simulink model "sync_mach_disc_sim"  (R2017a)
settings: Solver=FixedStepAuto  StartTime=0.0  StopTime=10.0  FixedStep=1e-5  RelTol=1e-3
values from neighbouring files (symbols this model uses):
  L_1 = inv(L)    [smparamlib.m]
  Ra = .018    (= 0.018)    [smparamlib.m]
  Rf = 0.001    [smparamlib.m]
  Rkd = 0.02    [smparamlib.m]
  Rkq = 0.04    [smparamlib.m]
  wo = 2*pi*freq0    (= 376.991118431)    [smparamlib.m]
undefined symbols (not defined in the file or in its folder): DiscIntNeverNeededParam
settings Model: Creator=krovchen  LastModifiedBy=krovchen
settings OptimizationCC: DefaultParameterBehavior=Inlined  UseDivisionForNetSlopeComputation=on  UseFloatMulNetSlope=on  InlineInvariantSignals=on  PassReuseOutputArgsAs=Individual arguments  ZeroExternalMemoryAtStartup=off  ZeroInternalMemoryAtStartup=off  NoFixptDivByZeroProtection=on  EfficientFloat2IntCast=on
settings DebuggingCC: ParameterTunabilityLossMsg=error
settings SFSimCC: MATLABDynamicMemAlloc=off
settings RTWCC: SystemTargetFile=ert.tlc  GenCodeOnly=on  GenerateMakefile=off  PackageGeneratedCodeAndArtifacts=on  PackageName=v1_model_export  TemplateMakefile=RTW.MSVCBuild  Description=Create Visual C/C++ Solution File for Embedded Coder  GenerateReport=on  IncludeHyperlinkInReport=on  LaunchReport=on  TargetLang=C++  GenerateTraceInfo=on  GenerateTraceReport=on  GenerateTraceReportSl=on  GenerateTraceReportSf=on  GenerateTraceReportEml=on
settings CodeAppCC: ForceParamTrailComments=on  IgnoreCustomStorageClasses=off  OperatorAnnotations=on  SimulinkDataObjDesc=on  SFDataObjDesc=on  MATLABFcnDesc=on  CustomSymbolStrGlobalVar=rt$N$M  CustomSymbolStrType=$N$M  CustomSymbolStrFcn=$N$M$F  CustomSymbolStrMacro=$N$M  InsertBlockDesc=on  MATLABSourceComments=on
settings ERTTargetCC: TargetLangStandard=C++03 (ISO)  GenerateSampleERTMain=on  MultiInstanceERTCode=on  CodeInterfacePackaging=C++ class  SupportContinuousTime=on  InlinedParameterPlacement=NonHierarchical  RootIOFormat=Structure reference  ERTCustomFileTemplate=example_file_process.tlc

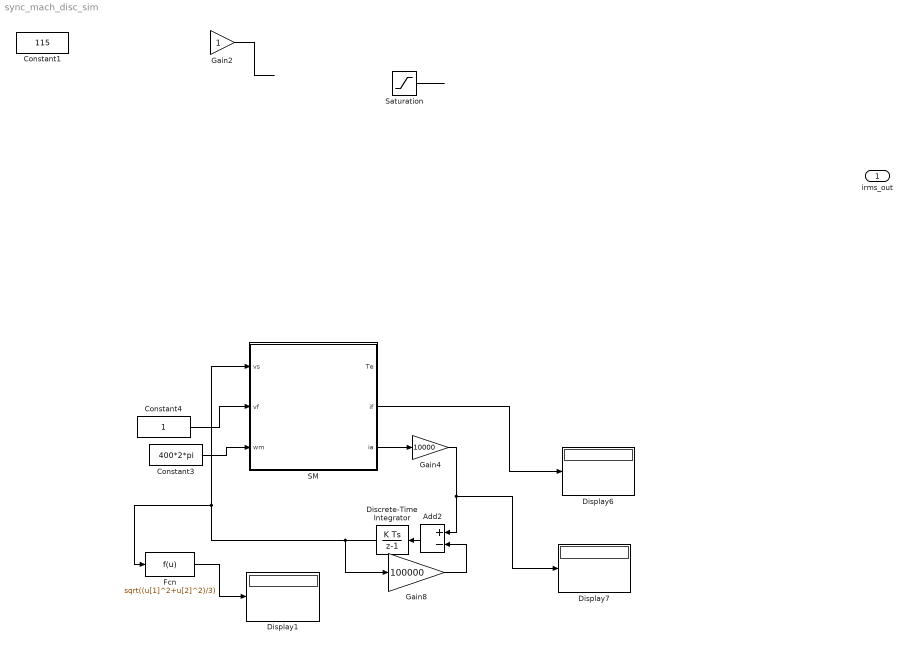
== system sync_mach_disc_sim ==
  Add2 : Sum  Inputs=+-
  Constant1 : Constant  Value=115
  Constant3 : Constant  Value=400*2*pi
  Constant4 : Constant
  Discrete-Time Integrator : DiscreteIntegrator  InitialConditionSetting=State (most efficient)  SampleTime=-1  ICPrevOutput=DiscIntNeverNeededParam  ICPrevScaledInput=DiscIntNeverNeededParam
  Display1 : Display
  Display6 : Display
  Display7 : Display
  Fcn : Fcn  Expr=sqrt((u[1]^2+u[2]^2)/3)
  Gain2 : Gain
  Gain4 : Gain  Gain=10000
  Gain8 : Gain  Gain=100000
  SM : Subsystem
      mask Display:
      | plot(-1.5,-1.5,1.5,1.5,cos(0:.01:7),sin(0:.01:7),[-.5 -1 1 .5],[-.866 -1.2 -1.2 -.866] )
      | disp('SYNCHRONOUS\nMACHINE')
  Saturation : Saturate  UpperLimit=1  LowerLimit=-1
  irms_out : Outport
  wires:
  ? -> ?
  ? -> Saturation/1
  Gain2/1 -> ?
  Saturation/1 -> ?
  Constant3/1 -> SM/3(wm)
  Constant4/1 -> SM/2(vf)
  SM/3(ia) -> Gain4/1
  Add2/1 -> Discrete-Time Integrator/1
  Gain4/1 -> Display7/1, Add2/1
  Discrete-Time Integrator/1 -> Gain8/1, Fcn/1, SM/1(vs)
  SM/2(if) -> Display6/1
  Gain8/1 -> Add2/2
  Fcn/1 -> Display1/1

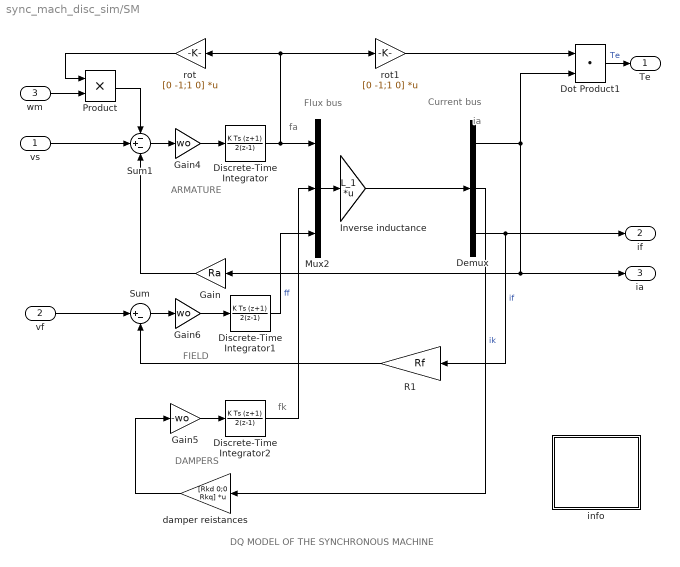
== system sync_mach_disc_sim/SM ==
  note: DAMPERS
  note: ARMATURE
  note: fa
  note: fk
  note: ia
  note: FIELD
  note: DQ MODEL OF THE SYNCHRONOUS MACHINE
  note: Flux bus
  note: Current bus
  vs : Inport
  vf : Inport  Port=2
  wm : Inport  Port=3
  Demux : Demux  Outputs=3
  Discrete-Time Integrator : DiscreteIntegrator  IntegratorMethod=Integration: Trapezoidal  InitialConditionSetting=State (most efficient)  SampleTime=-1  ICPrevOutput=DiscIntNeverNeededParam  ICPrevScaledInput=DiscIntNeverNeededParam
  Discrete-Time Integrator1 : DiscreteIntegrator  IntegratorMethod=Integration: Trapezoidal  InitialConditionSetting=State (most efficient)  SampleTime=-1  ICPrevOutput=DiscIntNeverNeededParam  ICPrevScaledInput=DiscIntNeverNeededParam
  Discrete-Time Integrator2 : DiscreteIntegrator  IntegratorMethod=Integration: Trapezoidal  InitialConditionSetting=State (most efficient)  SampleTime=-1  ICPrevOutput=DiscIntNeverNeededParam  ICPrevScaledInput=DiscIntNeverNeededParam
  Dot Product1 : DotProduct  InputSameDT=on  OutDataTypeStr=Inherit: Inherit via internal rule
  Gain : Gain  Gain=Ra  SaturateOnIntegerOverflow=on  OutDataTypeStr=Inherit: Same as input  ParamDataTypeStr=Inherit: Same as input
  Gain4 : Gain  Gain=wo  SaturateOnIntegerOverflow=on  OutDataTypeStr=Inherit: Same as input  ParamDataTypeStr=Inherit: Same as input
  Gain5 : Gain  Gain=-wo  SaturateOnIntegerOverflow=on  OutDataTypeStr=Inherit: Same as input  ParamDataTypeStr=Inherit: Same as input
  Gain6 : Gain  Gain=wo  SaturateOnIntegerOverflow=on  OutDataTypeStr=Inherit: Same as input  ParamDataTypeStr=Inherit: Same as input
  Inverse inductance : Gain  Gain=L_1  Multiplication=Matrix(K*u)  SaturateOnIntegerOverflow=on  OutDataTypeStr=Inherit: Same as input  ParamDataTypeStr=Inherit: Same as input
  Mux2 : Mux  Inputs=3
  Product : Product  SaturateOnIntegerOverflow=on  InputSameDT=on  OutDataTypeStr=Inherit: Same as first input
  R1 : Gain  Gain=Rf  SaturateOnIntegerOverflow=on  OutDataTypeStr=Inherit: Same as input  ParamDataTypeStr=Inherit: Same as input
  Sum : Sum  Inputs=|+-  SaturateOnIntegerOverflow=on  InputSameDT=on  OutDataTypeStr=Inherit: Same as first input
  Sum1 : Sum  Inputs=-+-  SaturateOnIntegerOverflow=on  InputSameDT=on  OutDataTypeStr=Inherit: Same as first input
  damper reistances : Gain  Gain=[Rkd 0;0 Rkq]  Multiplication=Matrix(K*u)  SaturateOnIntegerOverflow=on  OutDataTypeStr=Inherit: Same as input  ParamDataTypeStr=Inherit: Same as input
  info : Subsystem
      settings: OpenFcn=helpview(which('smeq0.htm'));
      mask Display:
      | plot(-1.5,-1.5,1.5,1.5,cos(0:.01:7),sin(0:.01:7) )
      | disp('Equations')
  rot : Gain  Gain=[0 -1;1 0]  Multiplication=Matrix(K*u)  SaturateOnIntegerOverflow=on  OutDataTypeStr=Inherit: Same as input  ParamDataTypeStr=Inherit: Same as input
  rot1 : Gain  Gain=[0 -1;1 0]  Multiplication=Matrix(K*u)  SaturateOnIntegerOverflow=on  OutDataTypeStr=Inherit: Same as input  ParamDataTypeStr=Inherit: Same as input
  Te : Outport
  if : Outport  Port=2
  ia : Outport  Port=3
  wires:
  Product/1 -> Sum1/1
  rot/1 -> Product/1
  wm/1 -> Product/2
  Gain5/1 -> Discrete-Time Integrator2/1
  damper reistances/1 -> Gain5/1
  Discrete-Time Integrator/1 -> Mux2/1, rot/1, rot1/1
  Sum1/1 -> Gain4/1
  Gain4/1 -> Discrete-Time Integrator/1
  vs/1 -> Sum1/2
  Gain/1 -> Sum1/3
  Gain6/1 -> Discrete-Time Integrator1/1
  Sum/1 -> Gain6/1
  vf/1 -> Sum/1
  rot1/1 -> Dot Product1/1
  Dot Product1/1 -> Te/1  "Te"
  Mux2/1 -> Inverse inductance/1
  Discrete-Time Integrator2/1 -> Mux2/2
  Discrete-Time Integrator1/1 -> Mux2/3  "ff"
  Demux/3 -> if/1, R1/1  "if"
  Demux/2 -> damper reistances/1  "ik"
  Inverse inductance/1 -> Demux/1
  Demux/1 -> Gain/1, ia/1, Dot Product1/2
  R1/1 -> Sum/2

== system sync_mach_disc_sim/SM/info ==
  note: This  demonstration  illustrates  the dynamics of a synchronous generator, initially
      | at no load,  following a three-phase short circuit at the terminals.
  note: Synchronous machine transients
      | under shortcircuit
